simulink model "UseCase_v5_predictive"  (R2024b)
settings: Solver=ode1  StartTime=0.0  StopTime=365*24  FixedStep=0.2  RelTol=1e-3
undefined symbols (not defined in the file): rain_data
libraries: filter_lib x5, Harvester_lib x3, buffer_lib x3, Demand_lib x2, storage_lib x2, transport_lib x1
settings Model: SimulationMode=accelerator  Creator=marcv  LastModifiedBy=mvseg
settings RTWCC: GPUComputeCapability=3.5

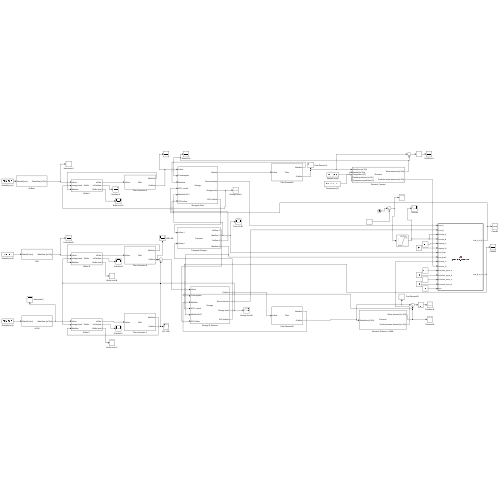
[thumbnail: Simulink's stored preview of the top-level diagram]
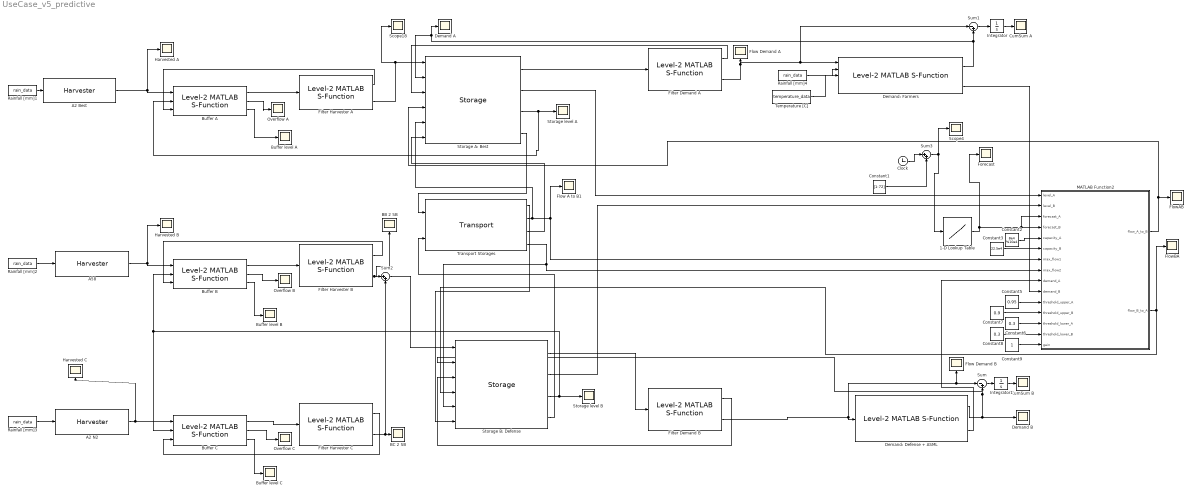
== system UseCase_v5_predictive ==
  1-D Lookup Table : Lookup_n-D  NumberOfTableDimensions=1  BreakpointsForDimension1=[0:8783]  Table=rain_data(:,2)  InternalRulePriority=Speed  RndMeth=Simplest
  A2 Best : Harvester_lib/Harvester  Type_harvester=Dependant on ground water (tunnel)  inflow_groundwater=91  Area=64000
  A2 N2 : Harvester_lib/Harvester  Type_harvester=Independant on ground water (resevoir, road ect.)  inflow_groundwater=1  Area=21e4
  A58 : Harvester_lib/Harvester  Type_harvester=Independant on ground water (resevoir, road ect.)  inflow_groundwater=1  Area=13.5e4
  BB 2 SB : Scope
  BC 2 SB : Scope
  Buffer A : buffer_lib/Level-2 MATLAB S-Function  Parameter1=2e4
  Buffer B : buffer_lib/Level-2 MATLAB S-Function  Parameter1=7e3
  Buffer C : buffer_lib/Level-2 MATLAB S-Function  Parameter1=1e4
  Buffer level A : Scope
  Buffer level B : Scope
  Buffer level C : Scope
  Clock : Clock
  Constant1 : Constant  Value=[1:72]
  Constant2 : Constant  Value=8e4 %10e4
  Constant3 : Constant  Value=22.5e4
  Constant5 : Constant  Value=0.95
  Constant6 : Constant  Value=0.3
  Constant7 : Constant  Value=0.9
  Constant8 : Constant  Value=0.3
  Constant9 : Constant
  CumSum A : Scope
  CumSum B : Scope
  Demand A : Scope
  Demand B : Scope
  Demand: Defense + ASML : Demand_lib/Level-2 MATLAB S-Function  Type_demand=Constant demand  Constant_demand=7e5  Crop_type=Potato  Area=8.5e5  Type_soil=Clay soil  Type_control=Predictive control  Predictive_steps=5
  Demand: Farmers : Demand_lib/Level-2 MATLAB S-Function  Type_demand=Agriculture  Constant_demand=6e5  Crop_type=Potato  Area=5e5  Type_soil=Clay soil  Type_control=Predictive control  Predictive_steps=72
  Filter Demand A : filter_lib/Level-2 MATLAB S-Function  filteroption=Custom filter  Parameter4=Cyclone-sand-UV [90 m3/h]  Parameter1=400  Parameter2=1
  Filter Demand B : filter_lib/Level-2 MATLAB S-Function  filteroption=Custom filter  Parameter4=Cyclone-sand-UV [90 m3/h]  Parameter1=100  Parameter2=1
  Filter Harvester A : filter_lib/Level-2 MATLAB S-Function  filteroption=Custom filter  Parameter4=Cyclone-sand-UV [90 m3/h]  Parameter1=200  Parameter2=1
  Filter Harvester B : filter_lib/Level-2 MATLAB S-Function  filteroption=Custom filter  Parameter4=Cyclone-sand-UV [90 m3/h]  Parameter1=100  Parameter2=1
  Filter Harvester C : filter_lib/Level-2 MATLAB S-Function  filteroption=Custom filter  Parameter4=Cyclone-sand-UV [90 m3/h]  Parameter1=100  Parameter2=1
  Flow A to B1 : Scope
  Flow Demand A : Scope
  Flow Demand B : Scope
  FlowAB : Scope
  FlowBA : Scope
  Forecast : Scope
  Harvested A : Scope
  Harvested B : Scope
  Harvested C : Scope
  Integrator : Integrator
  Integrator1 : Integrator
  MATLAB Function2 : MATLAB Function  TreatAsAtomicUnit=on
  Overflow A : Scope
  Overflow B : Scope
  Overflow C : Scope
  Rainfall [mm]{1..4} (4 alike) : FromWorkspace  VariableName=rain_data  OutDataTypeStr=double  SampleTime=1
  Scope18 : Scope
  Scope4 : Scope
  Storage A: Best : storage_lib/Storage  Parameter1=8e4 %10e4  Parameter2=0.8  Parameter3=1 interconnection
  Storage B: Defense : storage_lib/Storage  Parameter1=22.5e4  Parameter2=0.5  Parameter3=1 interconnection
  Storage level A : Scope
  Storage level B : Scope
  Sum : Sum  Inputs=|-+
  Sum1 : Sum  Inputs=|-+
  Sum2 : Sum  Inputs=|++
  Sum3 : Sum  Inputs=|++
  Temperature [C] : FromWorkspace  VariableName=temperature_data  OutDataTypeStr=double  SampleTime=1
  Transport Storages : transport_lib/Transport  max_flow_result1=200  max_flow_result2=200  flowDirec=Bidirectional  setupopt=Transport only  Transporttype=Custom  Dist=210  elevation=1  width=1  depth=1  diameter=1  dP=2  customflow=200  filteroption=Common filter  Fflowmax=0  dPfilter=0  selectedfilter=Sand [90 m3/h (UDI 4U4604)]  filterparallel=1
  wires:
  Rainfall [mm]1/1 -> A2 Best/1
  A2 Best/1 -> Buffer A/1, Harvested A/1
  Buffer A/3 -> Buffer level A/1
  Filter Harvester A/1 -> Buffer A/3
  Buffer A/1 -> Filter Harvester A/1
  Buffer A/2 -> Overflow A/1
  Filter Harvester A/2 -> Storage A: Best/1, Scope18/1
  Storage A: Best/1 -> Filter Demand A/1
  Storage A: Best/3 -> Buffer A/2, Storage level A/1
  Storage B: Defense/3 -> Storage level B/1, Buffer C/2, Buffer B/2
  Buffer B/2 -> Overflow B/1
  Buffer B/1 -> Filter Harvester B/1
  Filter Harvester B/1 -> Buffer B/3
  A58/1 -> Buffer B/1, Harvested B/1
  Buffer B/3 -> Buffer level B/1
  Rainfall [mm]2/1 -> A58/1
  Demand: Farmers/1 -> Storage A: Best/2, Demand A/1, Sum1/2
  Demand: Defense + ASML/1 -> Storage B: Defense/2, Sum/2, Demand B/1
  Storage B: Defense/1 -> Filter Demand B/1
  Rainfall [mm]4/1 -> Demand: Farmers/2
  Sum1/1 -> Integrator/1
  Integrator/1 -> CumSum A/1
  Integrator1/1 -> CumSum B/1
  Sum/1 -> Integrator1/1
  Filter Harvester C/1 -> Buffer C/3
  Buffer C/2 -> Overflow C/1
  Rainfall [mm]3/1 -> A2 N2/1
  Buffer C/1 -> Filter Harvester C/1
  Buffer C/3 -> Buffer level C/1
  A2 N2/1 -> Buffer C/1, Harvested C/1
  Filter Harvester B/2 -> BB 2 SB/1, Sum2/1
  Sum2/1 -> Storage B: Defense/1
  Filter Harvester C/2 -> BC 2 SB/1, Sum2/2
  Filter Demand A/1 -> Storage A: Best/3
  Filter Demand A/2 -> Flow Demand A/1, Sum1/1, Demand: Farmers/1
  Filter Demand B/2 -> Sum/1, Flow Demand B/1, Demand: Defense + ASML/1
  Filter Demand B/1 -> Storage B: Defense/3
  Transport Storages/4 -> MATLAB Function2/8(max_flow2), Storage B: Defense/5
  Storage A: Best/4 -> Transport Storages/1
  Transport Storages/1 -> Storage B: Defense/6
  Storage B: Defense/4 -> Transport Storages/2
  Transport Storages/3 -> Storage A: Best/6
  Temperature [C]/1 -> Demand: Farmers/3
  Demand: Farmers/2 -> MATLAB Function2/10(demand_B)
  Demand: Defense + ASML/2 -> MATLAB Function2/9(demand_A)
  Sum3/1 -> 1-D Lookup Table/1, Scope4/1
  1-D Lookup Table/1 -> Forecast/1, MATLAB Function2/4(forecast_B), MATLAB Function2/3(forecast_A)
  Constant1/1 -> Sum3/2
  Constant2/1 -> MATLAB Function2/5(capacity_A)
  Clock/1 -> Sum3/1
  Constant3/1 -> MATLAB Function2/6(capacity_B)
  Storage A: Best/2 -> MATLAB Function2/1(level_A)
  Transport Storages/2 -> Storage A: Best/5, MATLAB Function2/7(max_flow1), Flow A to B1/1
  Storage B: Defense/2 -> MATLAB Function2/2(level_B)
  MATLAB Function2/1(flow_A_to_B) -> FlowAB/1, Storage A: Best/4
  MATLAB Function2/2(flow_B_to_A) -> Storage B: Defense/4, FlowBA/1
  Constant5/1 -> MATLAB Function2/11(threshold_upper_A)
  Constant6/1 -> MATLAB Function2/13(threshold_lower_A)
  Constant7/1 -> MATLAB Function2/12(threshold_upper_B)
  Constant9/1 -> MATLAB Function2/15(gain)
  Constant8/1 -> MATLAB Function2/14(threshold_lower_B)

== matlab function UseCase_v5_predictive/MATLAB Function2 ==
  data: level_A input; level_B input; forecast_A input; flow_A_to_B output; forecast_B input; capacity_A input; capacity_B input; max_flow1 input; max_flow2 input; flow_B_to_A output; demand_A input; demand_B input; threshold_upper_A input; threshold_upper_B input; threshold_lower_A input; threshold_lower_B input; gain input
function [flow_A_to_B, flow_B_to_A] = ...
    predictive_controller(level_A, level_B, ...
                          forecast_A, forecast_B, ...
                          capacity_A, capacity_B, ...
                          max_flow1, max_flow2, demand_A, demand_B, threshold_upper_A, threshold_upper_B, threshold_lower_A, threshold_lower_B, gain)

    % threshold_upper_A = 0.8;
    % threshold_upper_B = 0.8;
    % threshold_lower_A = 0.2;
    % threshold_lower_B = 0.2;

    part_A = level_A/capacity_A;
    part_B = level_B/capacity_B;

    % gain = 1;

    predicted_A = zeros(72,1);
    predicted_B = zeros(72,1);

    % Compute threshold levels in m^3
    %threshold_level_A = threshold * capacity_A;
    %threshold_level_B = threshold * capacity_B;

    % Predict levels
    for i = 1:72
        predicted_A(i) = level_A + sum(forecast_A(1:i)) - i * demand_A;
        predicted_B(i) = level_B + sum(forecast_B(1:i)) - sum(demand_B(1:i));
    end

    % Get worst-case predicted levels
    max_predicted_A = max(predicted_A)/capacity_A;
    max_predicted_B = max(predicted_B)/capacity_B;

    min_predicted_A = min(predicted_A)/capacity_A;
    min_predicted_B = min(predicted_B)/capacity_B;

    % % Compute overflow amounts (above threshold)
    % overflow_A = max(max_predicted_A - threshold_level_A, 0);
    % overflow_B = max(max_predicted_B - threshold_level_B, 0);
    % 
    % % Safety check: do not allow transfer if the other tank would exceed threshold
    % will_A_overflow = max_predicted_A >= threshold_level_A;
    % will_B_overflow = max_predicted_B >= threshold_level_B;
    % 
    % % Define a buffer margin to scale flows (e.g. 10% of capacity)
    % bufferA = 0.9 * capacity_A;
    % bufferB = 0.9 * capacity_B;

    % Control logic
%     if overflow_A > 0 && ~will_B_overflow
%         % Proportional transfer from A → B
%         flow_A_to_B = min(max_flow1, max_flow1 * (overflow_A / bufferA));
%         flow_B_to_A = 0;
%     elseif overflow_B > 0 && ~will_A_overflow
%         % Proportional transfer from B → A
%         flow_B_to_A = min(max_flow1, max_flow1 * (overflow_B / bufferB));
%         flow_A_to_B = 0;
%     else
%         flow_A_to_B = 0;
%         flow_B_to_A = 0;
%     end
% end


if (max_predicted_A >= threshold_upper_A) && (max_predicted_B >= threshold_upper_B)
    if part_A > part_B
        flow_A_to_B = abs(min(gain*(part_A - part_B), 1) * max_flow1);
        flow_B_to_A = 0;
    elseif part_A < part_B
        flow_A_to_B = 0;
        flow_B_to_A = abs(min(gain*(part_B - part_A), 1) * max_flow1);  
    else
        flow_A_to_B = 0;
        flow_B_to_A = 0; 
    end

elseif (max_predicted_A >= threshold_upper_A) && (max_predicted_B < threshold_upper_B)
    flow_A_to_B = abs(min(gain*(part_A - part_B), 1) * max_flow1);
    flow_B_to_A = 0;

elseif (max_predicted_A < threshold_upper_A) && (max_predicted_B >= threshold_upper_B)
    flow_A_to_B = 0;
    flow_B_to_A = abs(min(gain*(part_B - part_A), 1) * max_flow1);

elseif (max_predicted_A < threshold_upper_A) && (max_predicted_B < threshold_upper_B)
    flow_A_to_B = 0;
    flow_B_to_A = 0;
    
    if (min_predicted_A < threshold_lower_A) && (min_predicted_B < threshold_lower_B)
        if part_A < part_B
            flow_A_to_B = 0;
            flow_B_to_A = abs(min(gain*(part_B - part_A), 1) * max_flow2);
        elseif part_B < part_A
            flow_A_to_B = abs(min(gain*(part_A - part_B), 1) * max_flow1);
            flow_B_to_A = 0;
        else
            flow_A_to_B = 0;
            flow_B_to_A = 0;
        end

    elseif (min_predicted_A < threshold_lower_A)
        flow_A_to_B = 0;
        flow_B_to_A = abs(min(gain*(part_B - part_A), 1) * max_flow2);

    elseif (min_predicted_B < threshold_lower_B)
        flow_A_to_B = abs(min(gain*(part_A - part_B), 1) * max_flow1);
        flow_B_to_A = 0;

    else
        flow_A_to_B = 0;
        flow_B_to_A = 0;
   end

else
    flow_A_to_B = 0;
    flow_B_to_A = 0;
end
   


end
